simulink model "gm_uz_pmsm_model_6LUT_pd"  (R2023a)
settings: Solver=FixedStepAuto  StartTime=0.0  StopTime=0.05  RelTol=1e-3
PreLoadFcn:
  | uz_pmsm_model_init_parameter
PostLoadFcn:
  | % Import the data from Excel for a lookup table
  | FluxMapData = readtable('C:\Users\Philipp\ultrazohm\ultrazohm_sw\ip_cores\uz_pmsm_model\FluxMapData_2023-05-26_13-07-57.csv');
  | % Row indices for lookup table
  | d_current_in_d_axis = FluxMapData(8:27,1:end);
  | % Column indices for lookup table
  | q_current_in_d_axis = FluxMapData(29:48,1:end);
  | % Output values for lookup table
  | d_Flux_d_axis = FluxMapData(50:69,1:end);
undefined symbols (not defined in the file or in its folder): d_current_d_Flux, d_current_q_Flux, entkopplung_dynamic, entkopplung_linear, entkopplung_static, Flux_d, Flux_q, friction_coefficient, inertia, k_i_d, k_p_d, k_p_q, Ki_Bo_d, Ki_Bo_q, Kp_Bo_d, Kp_Bo_q, L_d, L_q, Ldd, Ldq, Lqd, Lqq, parameter_nachfuerung, polepair, praediktion_entkopplung_nonlinear, psi_pm, q_current_d_Flux, q_current_q_Flux, R_1, simulate_mechanical, simulate_nonlinear_modell, simulate_open_loop, static_friction_torque, tau_sum, ts, ts_regler
libraries: hdlmdlgenlib x5, slpidlib x4
(part 1 of 2)
settings Model: Creator=ts  LastModifiedBy=Philipp
settings SolverCC: AlgebraicLoopSolver=TrustRegion  AutoInsertRateTranBlk=on
settings DataIOCC: LimitDataPoints=on  SaveOutput=off  SaveTime=off
settings OptimizationCC: BlockReduction=off  ConditionallyExecuteInputs=off  DefaultParameterBehavior=Inlined  LifeSpan=inf
settings DebuggingCC: AlgebraicLoopMsg=error  InheritedTsInSrcMsg=none  SingleTaskRateTransMsg=error  UnconnectedInputMsg=warning  UnconnectedOutputMsg=warning  UnconnectedLineMsg=warning  AllowSymbolicDim=off  StrictBusMsg=ErrorOnBusTreatedAsVector  SFUnexpectedBacktrackingDiag=warning  SFNoUnconditionalDefaultTransitionDiag=warning  SFExecutionAtInitializationDiag=none  ArithmeticOperatorsInVariantConditions=warning
settings HardwareCC: ProdBitPerPointer=32  ProdBitPerSizeT=32  ProdBitPerPtrDiffT=32  ProdLargestAtomicFloat=None  ProdIntDivRoundTo=Undefined  ProdEndianess=Unspecified  ProdWordSize=32  ProdHWDeviceType=ASIC/FPGA->ASIC/FPGA  ProdEqTarget=off
settings ModelReferenceCC: EnableRefExpFcnMdlSchedulingChecks=on
settings SFSimCC: SimUseLocalCustomCode=off  CustomCodeUndefinedFunction=UseInterfaceOnly
settings RTWCC: RTWUseLocalCustomCode=off  DLArmComputeVersion=19.05
settings CodeAppCC: StateflowObjectComments=on
settings GRTTargetCC: TargetLangStandard=C89/C90 (ANSI)
settings ConfigComp: CovScope=ReferencedModels  CovMetricSettings=dw  CovSaveCumulativeToWorkspaceVar=on  CovSaveSingleToWorkspaceVar=on  CovExternalEMLEnable=off  CovSFcnEnable=off

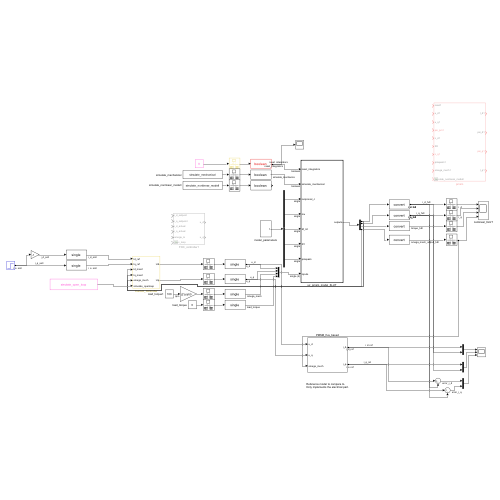
[thumbnail: Simulink's stored preview of the top-level diagram]
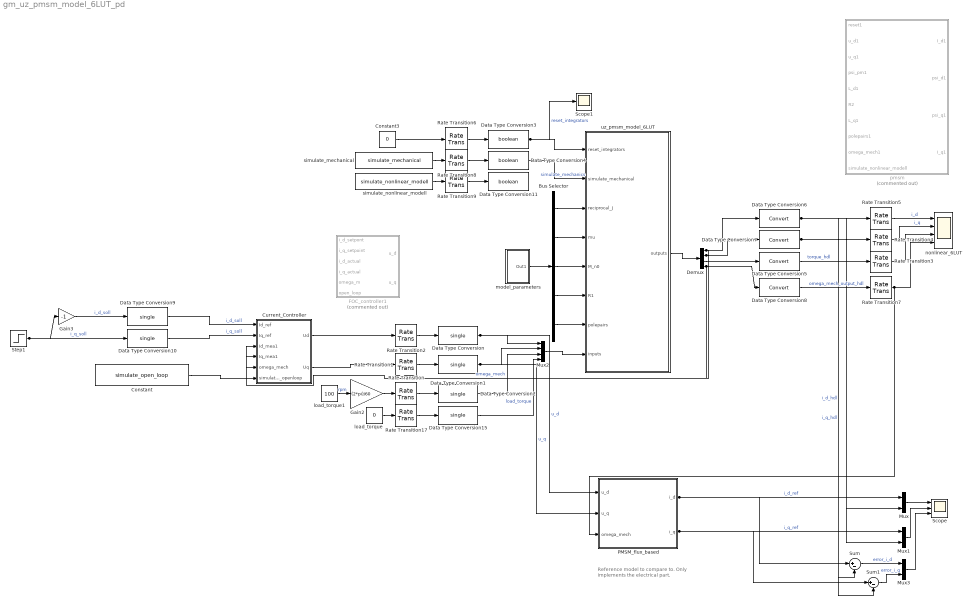
== system gm_uz_pmsm_model_6LUT_pd ==
  note: Reference model to compare to.
      | Only implements the electrical part.
  Bus Selector : BusSelector  OutputSignals=1_J,mu,M_R0,R_1,polepair
  Constant : Constant  Value=simulate_open_loop
  Constant3 : Constant  Value=0
  Current_Controller : Subsystem
  Data Type Conversion{,1..2,9..10,15} (6 alike) : DataTypeConversion  OutDataTypeStr=single  SaturateOnIntegerOverflow=off  RndMeth=Floor
  Data Type Conversion11 : DataTypeConversion  OutDataTypeStr=boolean  SaturateOnIntegerOverflow=off  RndMeth=Floor
  Data Type Conversion3 : DataTypeConversion  OutDataTypeStr=boolean  SaturateOnIntegerOverflow=off  RndMeth=Floor
  Data Type Conversion4 : DataTypeConversion  OutDataTypeStr=boolean  SaturateOnIntegerOverflow=off  RndMeth=Floor
  Data Type Conversion{5..8} (4 alike) : DataTypeConversion  SaturateOnIntegerOverflow=off  RndMeth=Floor
  Demux : Demux
  FOC_controller1 : Subsystem  Commented=on
  Gain2 : Gain  Gain=(2*pi)/60
  Gain3 : Gain  Gain=-1
  Mux : Mux  Inputs=2
  Mux1 : Mux  Inputs=2
  Mux2 : Mux
  Mux3 : Mux  Inputs=2
  PMSM_flux_based : Subsystem
  Rate Transition{,1..2,6,8..9,17} (7 alike) : RateTransition  OutPortSampleTime=ts
  Rate Transition{3..5,7} (4 alike) : RateTransition
  Scope : Scope  NumInputPorts=3
  Scope1 : Scope
  Step1 : Step  Time=0.025
  Sum : Sum  Inputs=|+-
  Sum1 : Sum  Inputs=|+-
  load_torque : Constant  Value=0
  load_torque1 : Constant  Value=100
  model_parameters : Subsystem
  nonlinear_6LUT : Scope  NumInputPorts=4
  pmsm : Subsystem  Commented=on
  simulate_mechanical : Constant  Value=simulate_mechanical
  simulate_nonlinear_modell : Constant  Value=simulate_nonlinear_modell
  uz_pmsm_model_6LUT : Subsystem  TreatAsAtomicUnit=on
  wires:
  Rate Transition9/1 -> Data Type Conversion11/1
  simulate_nonlinear_modell/1 -> Rate Transition9/1
  load_torque1/1 -> Gain2/1  "rpm"
  Constant/1 -> Current_Controller/6(simulate_openloop)
  Gain2/1 -> Rate Transition/1
  Current_Controller/2(Uq) -> Rate Transition1/1
  Current_Controller/1(Ud) -> Rate Transition2/1
  Data Type Conversion10/1 -> Current_Controller/2(Iq_ref)  "i_q_soll"
  Data Type Conversion9/1 -> Current_Controller/1(Id_ref)  "i_d_soll"
  uz_pmsm_model_6LUT/1(outputs) -> Demux/1
  Mux2/1 -> uz_pmsm_model_6LUT/8(inputs)
  Data Type Conversion2/1 -> Mux2/3  "omega_mech"
  Data Type Conversion15/1 -> Mux2/4  "load_torque"
  Data Type Conversion1/1 -> Mux2/2, PMSM_flux_based/2(u_q)  "u_q"
  Data Type Conversion/1 -> Mux2/1, PMSM_flux_based/1(u_d)  "u_d"
  Demux/2 -> Data Type Conversion7/1, Current_Controller/4(Iq_mea1)
  Demux/4 -> Data Type Conversion8/1, Current_Controller/5(omega_mech)
  Demux/1 -> Data Type Conversion6/1, Current_Controller/3(Id_mea1)
  Gain3/1 -> Data Type Conversion9/1  "i_d_soll"
  Demux/3 -> Data Type Conversion5/1
  Step1/1 -> Data Type Conversion10/1, Gain3/1  "i_q_soll"
  Mux3/1 -> Scope/3
  Sum1/1 -> Mux3/2  "error_i_q"
  Sum/1 -> Mux3/1  "error_i_d"
  model_parameters/1(Out1) -> Bus Selector/1
  Bus Selector/5 -> uz_pmsm_model_6LUT/7(polepairs)
  Bus Selector/4 -> uz_pmsm_model_6LUT/6(R1)
  Bus Selector/3 -> uz_pmsm_model_6LUT/5(M_n0)
  Bus Selector/2 -> uz_pmsm_model_6LUT/4(mu)
  Bus Selector/1 -> uz_pmsm_model_6LUT/3(reciprocal_J)
  Rate Transition7/1 -> nonlinear_6LUT/4, PMSM_flux_based/3(omega_mech)
  Data Type Conversion8/1 -> Rate Transition7/1  "omega_mech_output_hdl"
  PMSM_flux_based/1(i_d) -> Sum/1, Mux/1  "i_d_ref"
  PMSM_flux_based/2(i_q) -> Sum1/1, Mux1/1  "i_q_ref"
  Mux1/1 -> Scope/2
  Mux/1 -> Scope/1
  Rate Transition17/1 -> Data Type Conversion15/1
  load_torque/1 -> Rate Transition17/1
  Data Type Conversion4/1 -> uz_pmsm_model_6LUT/2(simulate_mechanical)  "simulate_mechanics"
  Data Type Conversion3/1 -> uz_pmsm_model_6LUT/1(reset_integrators), Scope1/1  "reset_integrators"
  simulate_mechanical/1 -> Rate Transition8/1
  Rate Transition8/1 -> Data Type Conversion4/1
  Constant3/1 -> Rate Transition6/1
  Rate Transition6/1 -> Data Type Conversion3/1
  Rate Transition3/1 -> nonlinear_6LUT/3
  Rate Transition5/1 -> nonlinear_6LUT/1  "i_d"
  Rate Transition4/1 -> nonlinear_6LUT/2  "i_q"
  Data Type Conversion5/1 -> Rate Transition3/1  "torque_hdl"
  Data Type Conversion7/1 -> Sum1/2, Mux1/2, Rate Transition4/1  "i_q_hdl"
  Data Type Conversion6/1 -> Rate Transition5/1, Sum/2, Mux/2  "i_d_hdl"
  Rate Transition2/1 -> Data Type Conversion/1
  Rate Transition1/1 -> Data Type Conversion1/1
  Rate Transition/1 -> Data Type Conversion2/1

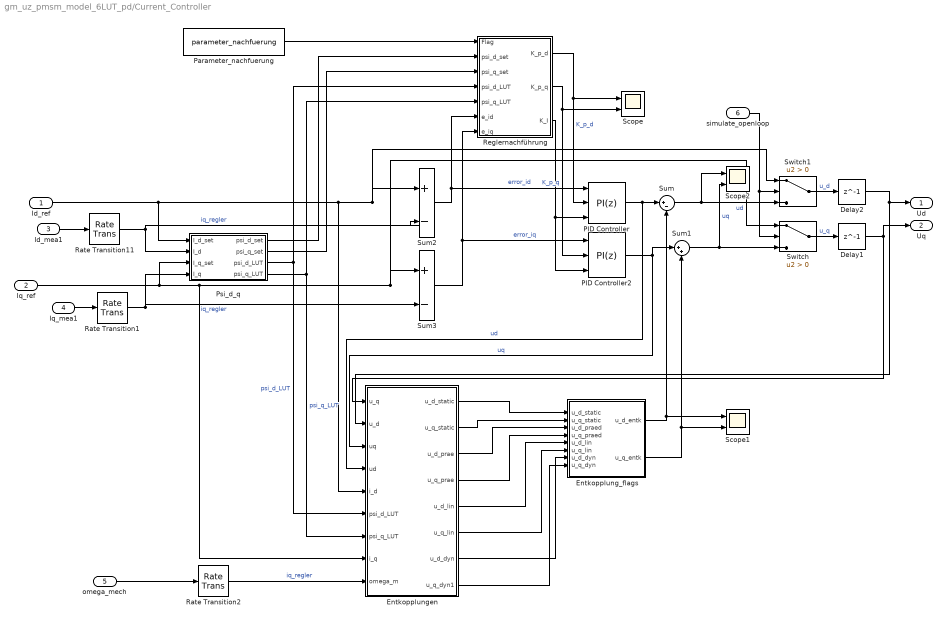
== system gm_uz_pmsm_model_6LUT_pd/Current_Controller ==
  Id_ref : Inport
  Iq_ref : Inport  Port=2
  Id_mea1 : Inport  Port=3
  Iq_mea1 : Inport  Port=4
  omega_mech : Inport  Port=5
  simulate_openloop : Inport  Port=6
  Delay1 : Delay  DelayLength=1
  Delay2 : Delay  DelayLength=1
  Entkopplung_flags : Subsystem
  Entkopplungen : Subsystem
  PID Controller : slpidlib/PID Controller  Controller=PI  Form=Parallel  TimeDomain=Discrete-time  UseExternalTs=off  SampleTime=-1  IntegratorMethod=Forward Euler  FilterMethod=Forward Euler  ControllerParametersSource=external  P=Kp_Bo_d  I=Ki_Bo_d  UseKiTs=off  D=0  N=100  UseFilter=on  TunerSelectOption=Transfer Function Based (PID Tuner App)  InitialConditionSource=internal  InitialConditionForIntegrator=0  InitialConditionForFilter=0  DifferentiatorICPrevScaledInput=0  ExternalReset=none  TrackingMode=off  Kt=1  LimitOutput=off  SatLimitsSource=internal  UpperSaturationLimit=48  LowerSaturationLimit=-48  LinearizeAsGain=off  AntiWindupMode=clamping  Kb=1  LimitIntegrator=off  UpperIntegratorSaturationLimit=48  LowerIntegratorSaturationLimit=-48  POutMin=[]  POutMax=[]  IOutMin=[]  IOutMax=[]  DOutMin=[]  DOutMax=[]  NOutMin=[]  NOutMax=[]  SumOutMin=[]  SumOutMax=[]  SaturationOutMin=[]  SaturationOutMax=[]  PParamMin=[]  PParamMax=[]  IParamMin=[]  IParamMax=[]  DParamMin=[]  DParamMax=[]  NParamMin=[]  NParamMax=[]  KbParamMin=[]  KbParamMax=[]  KtParamMin=[]  KtParamMax=[]  KbOutMin=[]  KbOutMax=[]  KtOutMin=[]  KtOutMax=[]  IntegratorOutMin=[]  IntegratorOutMax=[]  FilterOutMin=[]  FilterOutMax=[]  SumI1OutMin=[]  SumI1OutMax=[]  SumI2OutMin=[]  SumI2OutMax=[]  SumI3OutMin=[]  SumI3OutMax=[]  SumI4OutMin=[]  SumI4OutMax=[]  SumDOutMin=[]  SumDOutMax=[]  DifferentiatorOutMin=[]  DifferentiatorOutMax=[]  FilterDiffOutCoefMin=[]  FilterDiffOutCoefMax=[]  ReciprocalOutMin=[]  ReciprocalOutMax=[]  SumDenOutMin=[]  SumDenOutMax=[]  SumNumOutMin=[]  SumNumOutMax=[]  DivideOutMin=[]  DivideOutMax=[]  UdiffTsProdOutMin=[]  UdiffTsProdOutMax=[]  NTsProdOutMin=[]  NTsProdOutMax=[]  UintegralTsProdOutMin=[]  UintegralTsProdOutMax=[]  UngainTsProdOutMin=[]  UngainTsProdOutMax=[]  ClampingZeroOutDataTypeStr=Inherit: Inherit via back propagation  ClampingZeroOutMin=[]  ClampingZeroOutMax=[]  FilterDenConstantOutDataTypeStr=Inherit: Inherit via back propagation  FilterDenConstantOutMin=[]  FilterDenConstantOutMax=[]  PCopyOutDataTypeStr=Inherit: Inherit via back propagation  PCopyOutMin=[]  PCopyOutMax=[]  NCopyOutDataTypeStr=Inherit: Inherit via back propagation  NCopyOutMin=[]  NCopyOutMax=[]  IntegratorContinuousStateAttributes=''  IntegratorStateMustResolveToSignalObject=off  IntegratorRTWStateStorageClass=Auto  FilterContinuousStateAttributes=''  FilterStateMustResolveToSignalObject=off  FilterRTWStateStorageClass=Auto  ParallelPVariant=ExternalParameters  IdealPVariant=Disabled  IVariant=ExternalParameters  DVariant=Disabled  IntegratorVariant=Discrete  SatVariant=Disabled  AWVariant=Passthrough  PCopyVariant=Disabled  TRVariant=Disabled  FdbkBlocksVariant=Forward  IdealPFdbkVariant=Disabled  SatFdbkVariant=Disabled  DerivativeFilterVariant=Disabled  NVariant=Disabled  NCopyVariant=Disabled_SignalSpec  FilterICVariant=Disabled  IntegratorICVariant=InternalICs  ExternalResetVariant=Disabled  TRSumVariant=Passthrough  SumFdbkVariant=Disabled  SumVariant=Sum_PI  TsampFilterVariant=InternalTs  TsampNgainVariant=Passthrough  TsampIntegralVariant=Disabled_SignalSpec  ExternalSaturationOutDataTypeStr=Inherit: Same as second input
  PID Controller2 : slpidlib/PID Controller  Controller=PI  Form=Parallel  TimeDomain=Discrete-time  UseExternalTs=off  SampleTime=-1  IntegratorMethod=Forward Euler  FilterMethod=Forward Euler  ControllerParametersSource=external  P=Kp_Bo_q  I=Ki_Bo_q  UseKiTs=off  D=0  N=100  UseFilter=on  TunerSelectOption=Transfer Function Based (PID Tuner App)  InitialConditionSource=internal  InitialConditionForIntegrator=0  InitialConditionForFilter=0  DifferentiatorICPrevScaledInput=0  ExternalReset=none  TrackingMode=off  Kt=1  LimitOutput=off  SatLimitsSource=internal  UpperSaturationLimit=48  LowerSaturationLimit=-48  LinearizeAsGain=off  AntiWindupMode=clamping  Kb=1  LimitIntegrator=off  UpperIntegratorSaturationLimit=48  LowerIntegratorSaturationLimit=-48  POutMin=[]  POutMax=[]  IOutMin=[]  IOutMax=[]  DOutMin=[]  DOutMax=[]  NOutMin=[]  NOutMax=[]  SumOutMin=[]  SumOutMax=[]  SaturationOutMin=[]  SaturationOutMax=[]  PParamMin=[]  PParamMax=[]  IParamMin=[]  IParamMax=[]  DParamMin=[]  DParamMax=[]  NParamMin=[]  NParamMax=[]  KbParamMin=[]  KbParamMax=[]  KtParamMin=[]  KtParamMax=[]  KbOutMin=[]  KbOutMax=[]  KtOutMin=[]  KtOutMax=[]  IntegratorOutMin=[]  IntegratorOutMax=[]  FilterOutMin=[]  FilterOutMax=[]  SumI1OutMin=[]  SumI1OutMax=[]  SumI2OutMin=[]  SumI2OutMax=[]  SumI3OutMin=[]  SumI3OutMax=[]  SumI4OutMin=[]  SumI4OutMax=[]  SumDOutMin=[]  SumDOutMax=[]  DifferentiatorOutMin=[]  DifferentiatorOutMax=[]  FilterDiffOutCoefMin=[]  FilterDiffOutCoefMax=[]  ReciprocalOutMin=[]  ReciprocalOutMax=[]  SumDenOutMin=[]  SumDenOutMax=[]  SumNumOutMin=[]  SumNumOutMax=[]  DivideOutMin=[]  DivideOutMax=[]  UdiffTsProdOutMin=[]  UdiffTsProdOutMax=[]  NTsProdOutMin=[]  NTsProdOutMax=[]  UintegralTsProdOutMin=[]  UintegralTsProdOutMax=[]  UngainTsProdOutMin=[]  UngainTsProdOutMax=[]  ClampingZeroOutDataTypeStr=Inherit: Inherit via back propagation  ClampingZeroOutMin=[]  ClampingZeroOutMax=[]  FilterDenConstantOutDataTypeStr=Inherit: Inherit via back propagation  FilterDenConstantOutMin=[]  FilterDenConstantOutMax=[]  PCopyOutDataTypeStr=Inherit: Inherit via back propagation  PCopyOutMin=[]  PCopyOutMax=[]  NCopyOutDataTypeStr=Inherit: Inherit via back propagation  NCopyOutMin=[]  NCopyOutMax=[]  IntegratorContinuousStateAttributes=''  IntegratorStateMustResolveToSignalObject=off  IntegratorRTWStateStorageClass=Auto  FilterContinuousStateAttributes=''  FilterStateMustResolveToSignalObject=off  FilterRTWStateStorageClass=Auto  ParallelPVariant=ExternalParameters  IdealPVariant=Disabled  IVariant=ExternalParameters  DVariant=Disabled  IntegratorVariant=Discrete  SatVariant=Disabled  AWVariant=Passthrough  PCopyVariant=Disabled  TRVariant=Disabled  FdbkBlocksVariant=Forward  IdealPFdbkVariant=Disabled  SatFdbkVariant=Disabled  DerivativeFilterVariant=Disabled  NVariant=Disabled  NCopyVariant=Disabled_SignalSpec  FilterICVariant=Disabled  IntegratorICVariant=InternalICs  ExternalResetVariant=Disabled  TRSumVariant=Passthrough  SumFdbkVariant=Disabled  SumVariant=Sum_PI  TsampFilterVariant=InternalTs  TsampNgainVariant=Passthrough  TsampIntegralVariant=Disabled_SignalSpec  ExternalSaturationOutDataTypeStr=Inherit: Same as second input
  Parameter_nachfuerung : Constant  Value=parameter_nachfuerung
  Psi_d_q : Subsystem
  Rate Transition1 : RateTransition  OutPortSampleTime=ts_regler
  Rate Transition11 : RateTransition  OutPortSampleTime=ts_regler
  Rate Transition2 : RateTransition  OutPortSampleTime=ts_regler
  Reglernachführung : Subsystem
  Scope : Scope  NumInputPorts=2
  Scope1 : Scope  NumInputPorts=2
  Scope2 : Scope  NumInputPorts=2
  Sum : Sum  Inputs=|+-
  Sum1 : Sum  Inputs=|++
  Sum2 : Sum  Inputs=|+-
  Sum3 : Sum  Inputs=|+-
  Switch : Switch  Criteria=u2 > Threshold  SaturateOnIntegerOverflow=off  InputSameDT=off
  Switch1 : Switch  Criteria=u2 > Threshold  SaturateOnIntegerOverflow=off  InputSameDT=off
  Ud : Outport
  Uq : Outport  Port=2
  wires:
  Entkopplungen/8(u_q_dyn1) -> Entkopplung_flags/8(u_q_dyn)
  Entkopplungen/7(u_d_dyn) -> Entkopplung_flags/7(u_d_dyn)
  Delay1/1 -> Entkopplungen/1(u_q), Uq/1
  Delay2/1 -> Entkopplungen/2(u_d), Ud/1
  Rate Transition2/1 -> Entkopplungen/9(omega_m)  "iq_regler"
  Rate Transition1/1 -> Psi_d_q/4(I_q), Sum3/2  "iq_regler"
  Rate Transition11/1 -> Psi_d_q/2(I_d), Sum2/2  "iq_regler"
  Entkopplung_flags/2(u_q_entk) -> Sum1/2, Scope1/2
  Entkopplung_flags/1(u_d_entk) -> Sum/2, Scope1/1
  Entkopplungen/6(u_q_lin) -> Entkopplung_flags/6(u_q_lin)
  Entkopplungen/5(u_d_lin) -> Entkopplung_flags/5(u_d_lin)
  Entkopplungen/4(u_q_prae) -> Entkopplung_flags/4(u_q_praed)
  Entkopplungen/3(u_d_prae) -> Entkopplung_flags/3(u_d_praed)
  Entkopplungen/2(u_q_static) -> Entkopplung_flags/2(u_q_static)
  Entkopplungen/1(u_d_static) -> Entkopplung_flags/1(u_d_static)
  omega_mech/1 -> Rate Transition2/1
  Psi_d_q/2(psi_q_set) -> Reglernachführung/3(psi_q_set)
  Psi_d_q/1(psi_d_set) -> Reglernachführung/2(psi_d_set)
  Parameter_nachfuerung/1 -> Reglernachführung/1(Flag)
  Psi_d_q/4(psi_q_LUT) -> Entkopplungen/7(psi_q_LUT), Reglernachführung/5(psi_q_LUT)  "psi_q_LUT"
  Psi_d_q/3(psi_d_LUT) -> Entkopplungen/6(psi_d_LUT), Reglernachführung/4(psi_d_LUT)  "psi_d_LUT"
  Iq_mea1/1 -> Rate Transition1/1
  Id_mea1/1 -> Rate Transition11/1
  Reglernachführung/3(K_I) -> PID Controller/3, PID Controller2/3
  Reglernachführung/2(K_p_q) -> Scope/2, PID Controller2/2  "K_p_q"
  Reglernachführung/1(K_p_d) -> Scope/1, PID Controller/2  "K_p_d"
  simulate_openloop/1 -> Switch1/2, Switch/2
  Switch1/1 -> Delay2/1  "u_d"
  Switch/1 -> Delay1/1  "u_q"
  Id_ref/1 -> Switch1/1, Sum2/1, Entkopplungen/5(i_d), Psi_d_q/1(I_d_set)
  Iq_ref/1 -> Psi_d_q/3(I_q_set), Switch/1, Sum3/1, Entkopplungen/8(i_q)
  Sum1/1 -> Switch/3, Scope2/2  "uq"
  PID Controller2/1 -> Entkopplungen/3(uq), Sum1/1  "uq"
  PID Controller/1 -> Sum/1, Entkopplungen/4(ud)  "ud"
  Sum/1 -> Switch1/3, Scope2/1  "ud"
  Sum2/1 -> Reglernachführung/6(e_id), PID Controller/1  "error_id"
  Sum3/1 -> PID Controller2/1, Reglernachführung/7(e_iq)  "error_iq"

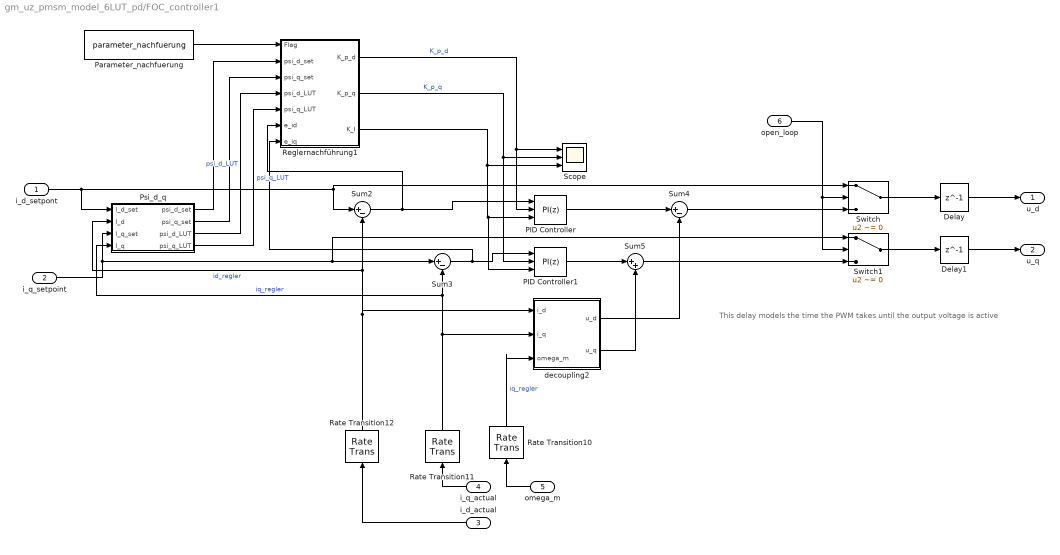
== system gm_uz_pmsm_model_6LUT_pd/FOC_controller1 ==
  note: This delay models the time the PWM takes until the output voltage is active
  i_d_setpont : Inport
  i_q_setpoint : Inport  Port=2
  i_d_actual : Inport  Port=3
  i_q_actual : Inport  Port=4
  omega_m : Inport  Port=5
  open_loop : Inport  Port=6
  Delay : Delay  DelayLength=1
  Delay1 : Delay  DelayLength=1
  PID Controller : slpidlib/PID Controller  Controller=PI  Form=Parallel  TimeDomain=Discrete-time  UseExternalTs=off  SampleTime=-1  IntegratorMethod=Forward Euler  FilterMethod=Forward Euler  ControllerParametersSource=external  P=k_p_d  I=k_i_d  UseKiTs=off  D=0  N=100  UseFilter=on  TunerSelectOption=Transfer Function Based (PID Tuner App)  InitialConditionSource=internal  InitialConditionForIntegrator=0  InitialConditionForFilter=0  DifferentiatorICPrevScaledInput=0  ExternalReset=none  TrackingMode=off  Kt=1  LimitOutput=off  SatLimitsSource=internal  UpperSaturationLimit=48  LowerSaturationLimit=-48  LinearizeAsGain=on  AntiWindupMode=clamping  Kb=1  LimitIntegrator=off  UpperIntegratorSaturationLimit=inf  LowerIntegratorSaturationLimit=-inf  POutMin=[]  POutMax=[]  IOutMin=[]  IOutMax=[]  DOutMin=[]  DOutMax=[]  NOutMin=[]  NOutMax=[]  SumOutMin=[]  SumOutMax=[]  SaturationOutMin=[]  SaturationOutMax=[]  PParamMin=[]  PParamMax=[]  IParamMin=[]  IParamMax=[]  DParamMin=[]  DParamMax=[]  NParamMin=[]  NParamMax=[]  KbParamMin=[]  KbParamMax=[]  KtParamMin=[]  KtParamMax=[]  KbOutMin=[]  KbOutMax=[]  KtOutMin=[]  KtOutMax=[]  IntegratorOutMin=[]  IntegratorOutMax=[]  FilterOutMin=[]  FilterOutMax=[]  SumI1OutMin=[]  SumI1OutMax=[]  SumI2OutMin=[]  SumI2OutMax=[]  SumI3OutMin=[]  SumI3OutMax=[]  SumI4OutMin=[]  SumI4OutMax=[]  SumDOutMin=[]  SumDOutMax=[]  DifferentiatorOutMin=[]  DifferentiatorOutMax=[]  FilterDiffOutCoefMin=[]  FilterDiffOutCoefMax=[]  ReciprocalOutMin=[]  ReciprocalOutMax=[]  SumDenOutMin=[]  SumDenOutMax=[]  SumNumOutMin=[]  SumNumOutMax=[]  DivideOutMin=[]  DivideOutMax=[]  UdiffTsProdOutMin=[]  UdiffTsProdOutMax=[]  NTsProdOutMin=[]  NTsProdOutMax=[]  UintegralTsProdOutMin=[]  UintegralTsProdOutMax=[]  UngainTsProdOutMin=[]  UngainTsProdOutMax=[]  ClampingZeroOutDataTypeStr=Inherit: Inherit via back propagation  ClampingZeroOutMin=[]  ClampingZeroOutMax=[]  FilterDenConstantOutDataTypeStr=Inherit: Inherit via back propagation  FilterDenConstantOutMin=[]  FilterDenConstantOutMax=[]  PCopyOutDataTypeStr=Inherit: Inherit via back propagation  PCopyOutMin=[]  PCopyOutMax=[]  NCopyOutDataTypeStr=Inherit: Inherit via back propagation  NCopyOutMin=[]  NCopyOutMax=[]  IntegratorContinuousStateAttributes=''  IntegratorStateMustResolveToSignalObject=off  IntegratorRTWStateStorageClass=Auto  FilterContinuousStateAttributes=''  FilterStateMustResolveToSignalObject=off  FilterRTWStateStorageClass=Auto  ParallelPVariant=ExternalParameters  IdealPVariant=Disabled  IVariant=ExternalParameters  DVariant=Disabled  IntegratorVariant=Discrete  SatVariant=Disabled  AWVariant=Passthrough  PCopyVariant=Disabled  TRVariant=Disabled  FdbkBlocksVariant=Forward  IdealPFdbkVariant=Disabled  SatFdbkVariant=Disabled  DerivativeFilterVariant=Disabled  NVariant=Disabled  NCopyVariant=Disabled_SignalSpec  FilterICVariant=Disabled  IntegratorICVariant=InternalICs  ExternalResetVariant=Disabled  TRSumVariant=Passthrough  SumFdbkVariant=Disabled  SumVariant=Sum_PI  TsampFilterVariant=InternalTs  TsampNgainVariant=Passthrough  TsampIntegralVariant=Disabled_SignalSpec  ExternalSaturationOutDataTypeStr=Inherit: Same as second input
  PID Controller1 : slpidlib/PID Controller  Controller=PI  Form=Parallel  TimeDomain=Discrete-time  UseExternalTs=off  SampleTime=-1  IntegratorMethod=Forward Euler  FilterMethod=Forward Euler  ControllerParametersSource=external  P=k_p_q  I=k_i_d  UseKiTs=off  D=0  N=100  UseFilter=on  TunerSelectOption=Transfer Function Based (PID Tuner App)  InitialConditionSource=internal  InitialConditionForIntegrator=0  InitialConditionForFilter=0  DifferentiatorICPrevScaledInput=0  ExternalReset=none  TrackingMode=off  Kt=1  LimitOutput=off  SatLimitsSource=internal  UpperSaturationLimit=48  LowerSaturationLimit=-48  LinearizeAsGain=on  AntiWindupMode=clamping  Kb=1  LimitIntegrator=off  UpperIntegratorSaturationLimit=inf  LowerIntegratorSaturationLimit=-inf  POutMin=[]  POutMax=[]  IOutMin=[]  IOutMax=[]  DOutMin=[]  DOutMax=[]  NOutMin=[]  NOutMax=[]  SumOutMin=[]  SumOutMax=[]  SaturationOutMin=[]  SaturationOutMax=[]  PParamMin=[]  PParamMax=[]  IParamMin=[]  IParamMax=[]  DParamMin=[]  DParamMax=[]  NParamMin=[]  NParamMax=[]  KbParamMin=[]  KbParamMax=[]  KtParamMin=[]  KtParamMax=[]  KbOutMin=[]  KbOutMax=[]  KtOutMin=[]  KtOutMax=[]  IntegratorOutMin=[]  IntegratorOutMax=[]  FilterOutMin=[]  FilterOutMax=[]  SumI1OutMin=[]  SumI1OutMax=[]  SumI2OutMin=[]  SumI2OutMax=[]  SumI3OutMin=[]  SumI3OutMax=[]  SumI4OutMin=[]  SumI4OutMax=[]  SumDOutMin=[]  SumDOutMax=[]  DifferentiatorOutMin=[]  DifferentiatorOutMax=[]  FilterDiffOutCoefMin=[]  FilterDiffOutCoefMax=[]  ReciprocalOutMin=[]  ReciprocalOutMax=[]  SumDenOutMin=[]  SumDenOutMax=[]  SumNumOutMin=[]  SumNumOutMax=[]  DivideOutMin=[]  DivideOutMax=[]  UdiffTsProdOutMin=[]  UdiffTsProdOutMax=[]  NTsProdOutMin=[]  NTsProdOutMax=[]  UintegralTsProdOutMin=[]  UintegralTsProdOutMax=[]  UngainTsProdOutMin=[]  UngainTsProdOutMax=[]  ClampingZeroOutDataTypeStr=Inherit: Inherit via back propagation  ClampingZeroOutMin=[]  ClampingZeroOutMax=[]  FilterDenConstantOutDataTypeStr=Inherit: Inherit via back propagation  FilterDenConstantOutMin=[]  FilterDenConstantOutMax=[]  PCopyOutDataTypeStr=Inherit: Inherit via back propagation  PCopyOutMin=[]  PCopyOutMax=[]  NCopyOutDataTypeStr=Inherit: Inherit via back propagation  NCopyOutMin=[]  NCopyOutMax=[]  IntegratorContinuousStateAttributes=''  IntegratorStateMustResolveToSignalObject=off  IntegratorRTWStateStorageClass=Auto  FilterContinuousStateAttributes=''  FilterStateMustResolveToSignalObject=off  FilterRTWStateStorageClass=Auto  ParallelPVariant=ExternalParameters  IdealPVariant=Disabled  IVariant=ExternalParameters  DVariant=Disabled  IntegratorVariant=Discrete  SatVariant=Disabled  AWVariant=Passthrough  PCopyVariant=Disabled  TRVariant=Disabled  FdbkBlocksVariant=Forward  IdealPFdbkVariant=Disabled  SatFdbkVariant=Disabled  DerivativeFilterVariant=Disabled  NVariant=Disabled  NCopyVariant=Disabled_SignalSpec  FilterICVariant=Disabled  IntegratorICVariant=InternalICs  ExternalResetVariant=Disabled  TRSumVariant=Passthrough  SumFdbkVariant=Disabled  SumVariant=Sum_PI  TsampFilterVariant=InternalTs  TsampNgainVariant=Passthrough  TsampIntegralVariant=Disabled_SignalSpec  ExternalSaturationOutDataTypeStr=Inherit: Same as second input
  Parameter_nachfuerung : Constant  Value=parameter_nachfuerung
  Psi_d_q : Subsystem
  Rate Transition10 : RateTransition  OutPortSampleTime=ts_regler
  Rate Transition11 : RateTransition  OutPortSampleTime=ts_regler
  Rate Transition12 : RateTransition  OutPortSampleTime=ts_regler
  Reglernachführung1 : Subsystem
  Scope : Scope  NumInputPorts=3
  Sum2 : Sum  Inputs=|+-
  Sum3 : Sum  Inputs=|+-
  Sum4 : Sum  Inputs=|+-
  Sum5 : Sum  Inputs=|++
  Switch : Switch  Criteria=u2 ~= 0  SaturateOnIntegerOverflow=off  InputSameDT=off
  Switch1 : Switch  Criteria=u2 ~= 0  SaturateOnIntegerOverflow=off  InputSameDT=off
  decoupling2 : Subsystem
  u_d : Outport
  u_q : Outport  Port=2
  wires:
  Parameter_nachfuerung/1 -> Reglernachführung1/1(Flag)
  Psi_d_q/4(psi_q_LUT) -> Reglernachführung1/5(psi_q_LUT)  "psi_q_LUT"
  Psi_d_q/3(psi_d_LUT) -> Reglernachführung1/4(psi_d_LUT)  "psi_d_LUT"
  Psi_d_q/2(psi_q_set) -> Reglernachführung1/3(psi_q_set)
  Psi_d_q/1(psi_d_set) -> Reglernachführung1/2(psi_d_set)
  Reglernachführung1/3(K_I) -> Scope/3, PID Controller/3, PID Controller1/3
  Reglernachführung1/2(K_p_q) -> Scope/2, PID Controller1/2  "K_p_q"
  Reglernachführung1/1(K_p_d) -> Scope/1, PID Controller/2  "K_p_d"
  Delay1/1 -> u_q/1
  Delay/1 -> u_d/1
  Switch1/1 -> Delay1/1
  Switch/1 -> Delay/1
  decoupling2/2(u_q) -> Sum5/2
  decoupling2/1(u_d) -> Sum4/2
  Rate Transition10/1 -> decoupling2/3(omega_m)  "iq_regler"
  open_loop/1 -> Switch/2, Switch1/2
  i_q_setpoint/1 -> Psi_d_q/3(I_q_set), Sum3/1, Switch1/1
  Rate Transition11/1 -> decoupling2/2(i_q), Psi_d_q/4(I_q), Sum3/2  "iq_regler"
  Rate Transition12/1 -> decoupling2/1(i_d), Sum2/2, Psi_d_q/2(I_d)  "id_regler"
  i_q_actual/1 -> Rate Transition11/1
  Sum3/1 -> PID Controller1/1, Reglernachführung1/7(e_iq)
  omega_m/1 -> Rate Transition10/1
  Sum5/1 -> Switch1/3
  Sum2/1 -> PID Controller/1, Reglernachführung1/6(e_id)
  i_d_setpont/1 -> Psi_d_q/1(I_d_set), Switch/1, Sum2/1
  i_d_actual/1 -> Rate Transition12/1
  Sum4/1 -> Switch/3
  PID Controller1/1 -> Sum5/1
  PID Controller/1 -> Sum4/1

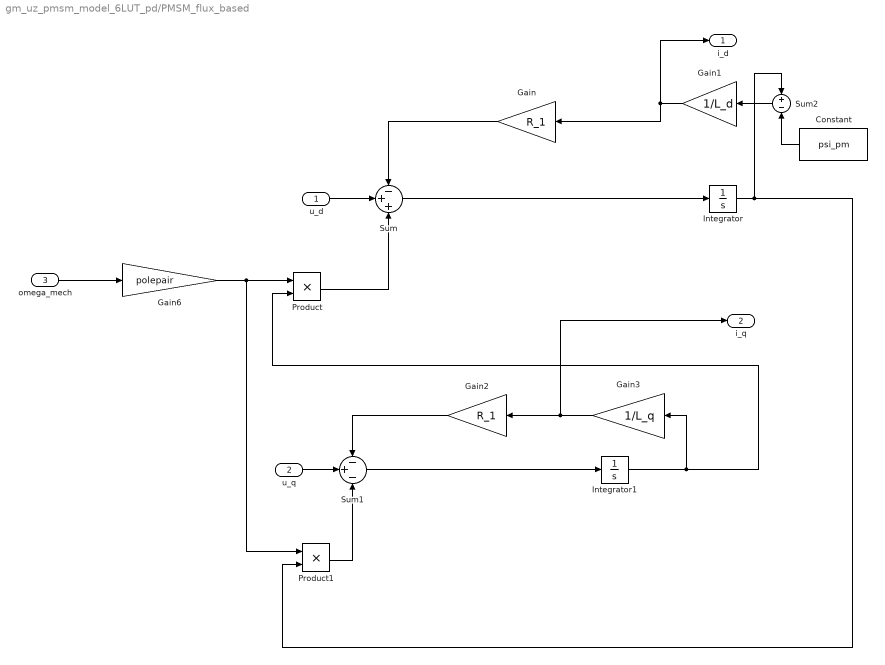
== system gm_uz_pmsm_model_6LUT_pd/PMSM_flux_based ==
  u_d : Inport
  u_q : Inport  Port=2
  omega_mech : Inport  Port=3
  Constant : Constant  Value=psi_pm
  Gain : Gain  Gain=R_1
  Gain1 : Gain  Gain=1/L_d
  Gain2 : Gain  Gain=R_1
  Gain3 : Gain  Gain=1/L_q
  Gain6 : Gain  Gain=polepair
  Integrator : Integrator
  Integrator1 : Integrator
  Product : Product
  Product1 : Product
  Sum : Sum  Inputs=-++
  Sum1 : Sum  Inputs=-+-
  Sum2 : Sum  Inputs=+-
  i_d : Outport
  i_q : Outport  Port=2
  wires:
  omega_mech/1 -> Gain6/1
  Gain3/1 -> Gain2/1, i_q/1
  Gain2/1 -> Sum1/1
  Sum1/1 -> Integrator1/1
  Product1/1 -> Sum1/3
  Integrator1/1 -> Product/2, Gain3/1
  Product/1 -> Sum/3
  Gain6/1 -> Product/1, Product1/1
  Gain1/1 -> i_d/1, Gain/1
  Sum2/1 -> Gain1/1
  Constant/1 -> Sum2/2
  Integrator/1 -> Sum2/1, Product1/2
  Gain/1 -> Sum/1
  Sum/1 -> Integrator/1
  u_q/1 -> Sum1/2
  u_d/1 -> Sum/2

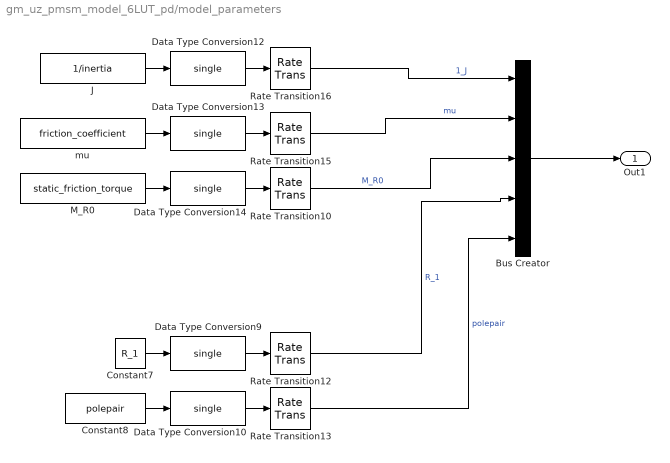
== system gm_uz_pmsm_model_6LUT_pd/model_parameters ==
  Bus Creator : BusCreator  Inputs=5
  Constant7 : Constant  Value=R_1
  Constant8 : Constant  Value=polepair
  Data Type Conversion{9..10,12..14} (5 alike) : DataTypeConversion  OutDataTypeStr=single  SaturateOnIntegerOverflow=off  RndMeth=Floor
  J : Constant  Value=1/inertia
  M_R0 : Constant  Value=static_friction_torque
  Rate Transition{10,12..13,15..16} (5 alike) : RateTransition  OutPortSampleTime=ts
  mu : Constant  Value=friction_coefficient
  Out1 : Outport
  wires:
  Constant7/1 -> Data Type Conversion9/1
  Data Type Conversion13/1 -> Rate Transition15/1
  M_R0/1 -> Data Type Conversion14/1
  mu/1 -> Data Type Conversion13/1
  Data Type Conversion10/1 -> Rate Transition13/1
  J/1 -> Data Type Conversion12/1
  Rate Transition15/1 -> Bus Creator/2  "mu"
  Data Type Conversion9/1 -> Rate Transition12/1
  Constant8/1 -> Data Type Conversion10/1
  Bus Creator/1 -> Out1/1
  Rate Transition13/1 -> Bus Creator/5  "polepair"
  Rate Transition16/1 -> Bus Creator/1  "1_J"
  Rate Transition12/1 -> Bus Creator/4  "R_1"
  Data Type Conversion14/1 -> Rate Transition10/1
  Rate Transition10/1 -> Bus Creator/3  "M_R0"
  Data Type Conversion12/1 -> Rate Transition16/1

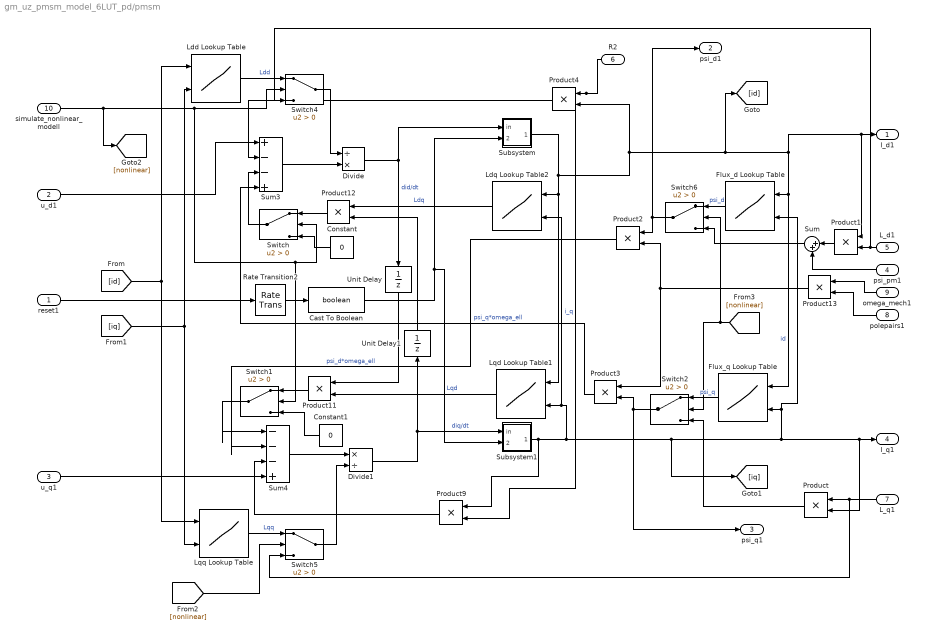
== system gm_uz_pmsm_model_6LUT_pd/pmsm ==
  reset1 : Inport
  u_d1 : Inport  Port=2
  u_q1 : Inport  Port=3
  psi_pm1 : Inport  Port=4
  L_d1 : Inport  Port=5
  R2 : Inport  Port=6
  L_q1 : Inport  Port=7
  polepairs1 : Inport  Port=8
  omega_mech1 : Inport  Port=9
  simulate_nonlinear_modell : Inport  Port=10
  Cast To Boolean : DataTypeConversion  OutDataTypeStr=boolean  SaturateOnIntegerOverflow=off  RndMeth=Floor
  Constant : Constant  Value=0  SampleTime=ts
  Constant1 : Constant  Value=0  SampleTime=ts
  Divide : Product  Inputs=/*
  Divide1 : Product  Inputs=*/
  Flux_d Lookup Table : Lookup_n-D  BreakpointsForDimension1=d_current_d_Flux  BreakpointsForDimension2=q_current_d_Flux  BreakpointsForDimension3=[5, 7]  Table=Flux_d  InternalRulePriority=Speed  RndMeth=Simplest
      settings: InputPortMap=u0,u1
  Flux_q Lookup Table : Lookup_n-D  BreakpointsForDimension1=d_current_q_Flux  BreakpointsForDimension2=q_current_q_Flux  BreakpointsForDimension3=[5, 7]  Table=Flux_q  InternalRulePriority=Speed  RndMeth=Simplest
      settings: InputPortMap=u0,u1
  Ldd Lookup Table : Lookup_n-D  BreakpointsForDimension1=d_current_q_Flux  BreakpointsForDimension2=q_current_q_Flux  BreakpointsForDimension3=[5, 7]  Table=Ldd  InternalRulePriority=Speed  RndMeth=Simplest
      settings: InputPortMap=u0,u1
  Ldq Lookup Table2 : Lookup_n-D  BreakpointsForDimension1=d_current_q_Flux  BreakpointsForDimension2=q_current_q_Flux  BreakpointsForDimension3=[5, 7]  Table=Ldq  InternalRulePriority=Speed  RndMeth=Simplest
      settings: InputPortMap=u0,u1
  Lqd Lookup Table1 : Lookup_n-D  BreakpointsForDimension1=d_current_q_Flux  BreakpointsForDimension2=q_current_q_Flux  BreakpointsForDimension3=[5, 7]  Table=Lqd  InternalRulePriority=Speed  RndMeth=Simplest
      settings: InputPortMap=u0,u1
  Lqq Lookup Table : Lookup_n-D  BreakpointsForDimension1=d_current_q_Flux  BreakpointsForDimension2=q_current_q_Flux  BreakpointsForDimension3=[5, 7]  Table=Lqq  InternalRulePriority=Speed  RndMeth=Simplest
      settings: InputPortMap=u0,u1
  Product{,1..4,9,11..13} (9 alike) : Product
  Rate Transition2 : RateTransition  OutPortSampleTime=ts
  Subsystem : Subsystem
  Subsystem1 : Subsystem
  Sum : Sum  Inputs=|++
  Sum3 : Sum  Inputs=|+--+
  Sum4 : Sum  Inputs=|---+
  Switch{,1..2,4..6} (6 alike) : Switch  Criteria=u2 > Threshold  SaturateOnIntegerOverflow=off  InputSameDT=off
  Unit Delay : UnitDelay  SampleTime=-1  HasFrameUpgradeWarning=on
  Unit Delay1 : UnitDelay  SampleTime=-1  HasFrameUpgradeWarning=on
  I_d1 : Outport
  psi_d1 : Outport  Port=2
  psi_q1 : Outport  Port=3
  I_q1 : Outport  Port=4
  wires:
  [nonlinear] -> Switch6/2, Switch2/2
  [nonlinear] -> Switch5/2
  simulate_nonlinear_modell/1 -> Switch4/2, Switch1/2, Switch/2, [nonlinear]
  Sum/1 -> Switch6/3
  Product1/1 -> Sum/1
  Switch6/1 -> Product2/1, psi_d1/1
  Flux_d Lookup Table/1 -> Switch6/1  "psi_d"
  Switch5/1 -> Divide1/2
  Lqq Lookup Table/1 -> Switch5/1  "Lqq"
  Switch4/1 -> Divide/1
  Ldd Lookup Table/1 -> Switch4/1  "Ldd"
  Product/1 -> Switch2/3
  Switch2/1 -> Product3/2, psi_q1/1
  Flux_q Lookup Table/1 -> Switch2/1  "psi_q"
  L_q1/1 -> Product/1, Switch5/3
  Constant1/1 -> Switch1/3
  Switch1/1 -> Sum4/1
  Product11/1 -> Switch1/1
  Constant/1 -> Switch/3
  Switch/1 -> Sum3/3
  Product12/1 -> Switch/1
  Ldq Lookup Table2/1 -> Product12/1  "Ldq"
  Lqd Lookup Table1/1 -> Product11/2  "Lqd"
  Unit Delay1/1 -> Product12/2
  Unit Delay/1 -> Product11/1
  Product2/1 -> Sum4/2  "psi_d*omega_ell"
  Product4/1 -> Sum3/2
  Product3/1 -> Sum3/4  "psi_q*omega_ell"
  [iq] -> Lqq Lookup Table/2, Ldd Lookup Table/2
  Subsystem1/1(outt) -> Product9/1, Lqd Lookup Table1/2, Ldq Lookup Table2/2, Flux_d Lookup Table/2, Flux_q Lookup Table/2, Product/2, I_q1/1, [iq]  "i_q"
  psi_pm1/1 -> Sum/2
  [id] -> Ldd Lookup Table/1, Lqq Lookup Table/1
  Subsystem/1(outt) -> [id], I_d1/1, Product1/1, Flux_q Lookup Table/1, Flux_d Lookup Table/1, Product4/2, Ldq Lookup Table2/1, Lqd Lookup Table1/1  "id"
  R2/1 -> Product4/1, Product9/2
  Rate Transition2/1 -> Cast To Boolean/1
  reset1/1 -> Rate Transition2/1
  u_d1/1 -> Sum3/1
  Cast To Boolean/1 -> Subsystem1/2(reset), Subsystem/2(reset)
  Product9/1 -> Sum4/3
  Sum3/1 -> Divide/2
  Divide/1 -> Subsystem/1(in), Unit Delay/1  "did/dt"
  Product13/1 -> Product2/2, Product3/1
  polepairs1/1 -> Product13/2
  Divide1/1 -> Subsystem1/1(in), Unit Delay1/1  "diq/dt"
  L_d1/1 -> Product1/2, Switch4/3
  omega_mech1/1 -> Product13/1
  u_q1/1 -> Sum4/4
  Sum4/1 -> Divide1/1

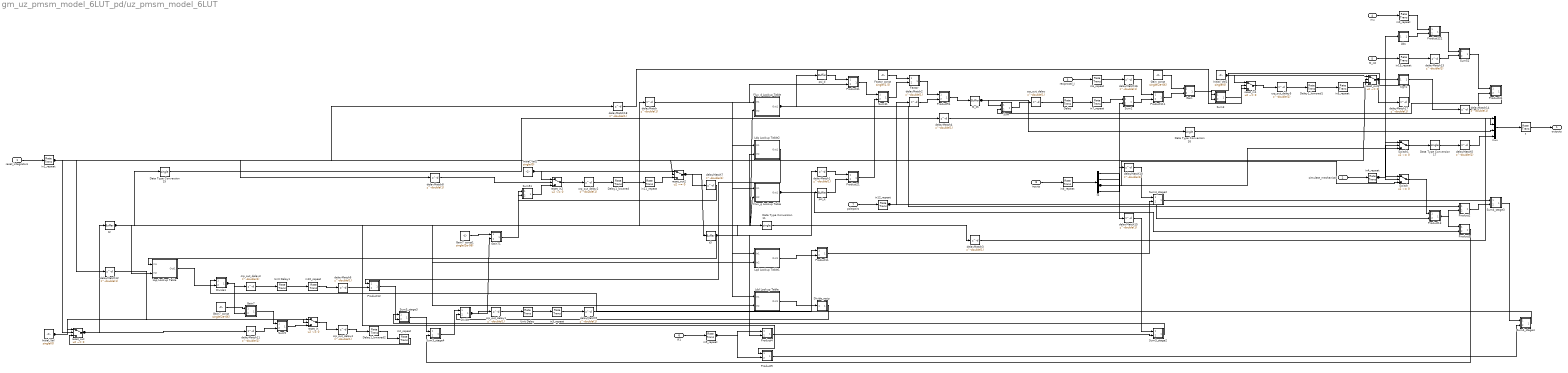
== system gm_uz_pmsm_model_6LUT_pd/uz_pmsm_model_6LUT ==
  reset_integrators : Inport  OutDataTypeStr=boolean  PortDimensions=1  SampleTime=2e-06
  simulate_mechanical : Inport  Port=2  OutDataTypeStr=boolean  PortDimensions=1  SampleTime=2e-06
  reciprocal_J : Inport  Port=3  OutDataTypeStr=single  PortDimensions=1  SampleTime=2e-06
  mu : Inport  Port=4  OutDataTypeStr=single  PortDimensions=1  SampleTime=2e-06
  M_n0 : Inport  Port=5  OutDataTypeStr=single  PortDimensions=1  SampleTime=2e-06
  R1 : Inport  Port=6  OutDataTypeStr=single  PortDimensions=1  SampleTime=2e-06
  polepairs : Inport  Port=7  OutDataTypeStr=single  PortDimensions=1  SampleTime=2e-06
  inputs : Inport  Port=8  OutDataTypeStr=single  PortDimensions=[4]  SampleTime=2e-06
  Abs : Subsystem
      mask Display: disp('NFP\nabs');
  Data Type Conversion{11,15..17} (4 alike) : DataTypeConversion  OutDataTypeStr=single
  Delay : RateTransition  OutPortSampleTimeOpt=Multiple of input port sample time  OutPortSampleTimeMultiple=200
  Delay1_lowered : RateTransition  OutPortSampleTimeOpt=Multiple of input port sample time  OutPortSampleTimeMultiple=200
  Delay1_lowered1 : RateTransition  OutPortSampleTimeOpt=Multiple of input port sample time  OutPortSampleTimeMultiple=200
  Delay1_lowered2 : RateTransition  OutPortSampleTimeOpt=Multiple of input port sample time  OutPortSampleTimeMultiple=200
  Divide : Subsystem
      mask Display: disp('NFP\nmul');
  Divide1 : Subsystem
      mask Display: disp('NFP\nmul');
  Divide_recip : Subsystem
      mask Display: disp('NFP\nmath');
  Factor : Subsystem
      mask Display: disp('NFP\nmul');
  Factor_const : Constant  Value=single(1.5)  OutDataTypeStr=single  SampleTime=1e-08
  Flux_d Lookup Table : Subsystem
  Flux_q Lookup Table : Subsystem
  Gain : Subsystem
      mask Display: disp('NFP\nmul');
  Gain7 : Subsystem
      mask Display: disp('NFP\nmul');
  Gain71 : Subsystem
      mask Display: disp('NFP\nmul');
  Gain7_const : Constant  Value=single(2e-06)  OutDataTypeStr=single  SampleTime=1e-08
  Gain7_const1 : Constant  Value=single(2e-06)  OutDataTypeStr=single  SampleTime=1e-08
  Gain_const : Constant  Value=single(2e-06)  OutDataTypeStr=single  SampleTime=1e-08
  Initial_Val : Constant  Value=single(0)  OutDataTypeStr=single  SampleTime=1e-08
  Initial_Val1 : Constant  Value=single(0)  OutDataTypeStr=single  SampleTime=1e-08
  Initial_Val2 : Constant  Value=single(0)  OutDataTypeStr=single  SampleTime=1e-08
  Ldd Lookup Table : Subsystem
  Ldq Lookup Table2 : Subsystem
  Lqd Lookup Table1 : Subsystem
  Lqq Lookup Table : Subsystem
  M_Mi : hdlmdlgenlib/Buffer
  Product11 : Subsystem
      mask Display: disp('NFP\nmul');
  Product111 : Subsystem
      mask Display: disp('NFP\nmul');
  Product12 : Subsystem
      mask Display: disp('NFP\nmul');
  Product121 : Subsystem
      mask Display: disp('NFP\nmul');
  Product13 : Subsystem
      mask Display: disp('NFP\nmul');
  Product2 : Subsystem
      mask Display: disp('NFP\nmul');
  Product21 : Subsystem
      mask Display: disp('NFP\nmul');
  Product3 : Subsystem
      mask Display: disp('NFP\nmul');
  Product31 : Subsystem
      mask Display: disp('NFP\nmul');
  Product4 : Subsystem
      mask Display: disp('NFP\nmul');
  Product41 : Subsystem
      mask Display: disp('NFP\nmul');
  Product9 : Subsystem
      mask Display: disp('NFP\nmul');
  Product91 : Subsystem
      mask Display: disp('NFP\nmul');
  Sign1 : Subsystem
      mask Display: disp('NFP\nsignum');
  Sum : Subsystem
      mask Display: disp('NFP\nadd');
  Sum1 : Subsystem
      mask Display: disp('NFP\nadd');
  Sum3 : Subsystem
      mask Display: disp('NFP\nadd');
  Sum31 : Subsystem
      mask Display: disp('NFP\nadd');
  Sum3_stage2 : Subsystem
      mask Display: disp('NFP\nadd');
  Sum3_stage3 : Subsystem
      mask Display: disp('NFP\nadd');
  Sum3_stage4 : Subsystem
      mask Display: disp('NFP\nadd');
  Sum4_stage2 : Subsystem
      mask Display: disp('NFP\nadd');
  Sum4_stage3 : Subsystem
      mask Display: disp('NFP\nadd');
  Sum4_stage4 : Subsystem
      mask Display: disp('NFP\nadd');
  Sum5 : Subsystem
      mask Display: disp('NFP\nadd');
  Sum51 : Subsystem
      mask Display: disp('NFP\nadd');
  Sum52 : Subsystem
      mask Display: disp('NFP\nadd');
  Switch : Switch  Criteria=u2 ~= 0  Threshold=double(0)  OutDataTypeStr=single  SampleTime=1e-08  SaturateOnIntegerOverflow=off  InputSameDT=off
  Switch1 : Switch  Criteria=u2 ~= 0  Threshold=double(0)  OutDataTypeStr=single  SampleTime=1e-08  SaturateOnIntegerOverflow=off  InputSameDT=off
  Unit Delay : RateTransition  OutPortSampleTimeOpt=Multiple of input port sample time  OutPortSampleTimeMultiple=200
  Unit Delay1 : RateTransition  OutPortSampleTimeOpt=Multiple of input port sample time  OutPortSampleTimeMultiple=200
  crp_out_delay{,1..5} (6 alike) : Delay  DelayLength=double(1)  InitialCondition=0  SampleTime=1e-08
  delayMatch{,1..18} (19 alike) : Delay  DelayLength=double(1)  InitialCondition=0  SampleTime=1e-08
  in0_repeat : RateTransition  Integrity=off  Deterministic=off  OutPortSampleTimeOpt=Multiple of input port sample time  OutPortSampleTimeMultiple=1/200
  in10_repeat : RateTransition  Integrity=off  Deterministic=off  OutPortSampleTimeOpt=Multiple of input port sample time  OutPortSampleTimeMultiple=1/200
  in11_repeat : RateTransition  Integrity=off  Deterministic=off  OutPortSampleTimeOpt=Multiple of input port sample time  OutPortSampleTimeMultiple=1/200
  in12_repeat : RateTransition  Integrity=off  Deterministic=off  OutPortSampleTimeOpt=Multiple of input port sample time  OutPortSampleTimeMultiple=1/200
  in13_repeat : RateTransition  Integrity=off  Deterministic=off  OutPortSampleTimeOpt=Multiple of input port sample time  OutPortSampleTimeMultiple=1/200
  in1_repeat : RateTransition  Integrity=off  Deterministic=off  OutPortSampleTimeOpt=Multiple of input port sample time  OutPortSampleTimeMultiple=1/200
  in2_repeat : RateTransition  Integrity=off  Deterministic=off  OutPortSampleTimeOpt=Multiple of input port sample time  OutPortSampleTimeMultiple=1/200
  in3_repeat : RateTransition  Integrity=off  Deterministic=off  OutPortSampleTimeOpt=Multiple of input port sample time  OutPortSampleTimeMultiple=1/200
  in4_repeat : RateTransition  Integrity=off  Deterministic=off  OutPortSampleTimeOpt=Multiple of input port sample time  OutPortSampleTimeMultiple=1/200
  in5_repeat : RateTransition  Integrity=off  Deterministic=off  OutPortSampleTimeOpt=Multiple of input port sample time  OutPortSampleTimeMultiple=1/200
  in6_repeat : RateTransition  Integrity=off  Deterministic=off  OutPortSampleTimeOpt=Multiple of input port sample time  OutPortSampleTimeMultiple=1/200
  in7_repeat : RateTransition  Integrity=off  Deterministic=off  OutPortSampleTimeOpt=Multiple of input port sample time  OutPortSampleTimeMultiple=1/200
  in8_repeat : RateTransition  Integrity=off  Deterministic=off  OutPortSampleTimeOpt=Multiple of input port sample time  OutPortSampleTimeMultiple=1/200
  in9_repeat : RateTransition  Integrity=off  Deterministic=off  OutPortSampleTimeOpt=Multiple of input port sample time  OutPortSampleTimeMultiple=1/200
  mux : Mux
  psi_d : hdlmdlgenlib/Buffer
  psi_q : hdlmdlgenlib/Buffer
  reset_in : Switch  Criteria=u2 ~= 0  Threshold=double(0)  OutDataTypeStr=single  SampleTime=1e-08  SaturateOnIntegerOverflow=off  InputSameDT=off
  reset_in1 : Switch  Criteria=u2 ~= 0  Threshold=double(0)  OutDataTypeStr=single  SampleTime=1e-08  SaturateOnIntegerOverflow=off  InputSameDT=off
  reset_in2 : Switch  Criteria=u2 ~= 0  Threshold=double(0)  OutDataTypeStr=single  SampleTime=1e-08  SaturateOnIntegerOverflow=off  InputSameDT=off
  reset_out : Switch  Criteria=u2 ~= 0  Threshold=double(0)  OutDataTypeStr=single  SampleTime=1e-08  SaturateOnIntegerOverflow=off  InputSameDT=off
  reset_out1 : Switch  Criteria=u2 ~= 0  Threshold=double(0)  OutDataTypeStr=single  SampleTime=1e-08  SaturateOnIntegerOverflow=off  InputSameDT=off
  reset_out2 : Switch  Criteria=u2 ~= 0  Threshold=double(0)  OutDataTypeStr=single  SampleTime=1e-08  SaturateOnIntegerOverflow=off  InputSameDT=off
  t : RateTransition  OutPortSampleTimeOpt=Multiple of input port sample time  OutPortSampleTimeMultiple=200
  t1 : Demux
  t2 : hdlmdlgenlib/Buffer
  t3 : hdlmdlgenlib/Buffer
  outputs : Outport  SampleTime=2e-06
  wires:
  reset_integrators/1 -> in1_repeat/1
  simulate_mechanical/1 -> in4_repeat/1
  reciprocal_J/1 -> in6_repeat/1
  mu/1 -> in0_repeat/1
  M_n0/1 -> in13_repeat/1
  R1/1 -> in9_repeat/1
  polepairs/1 -> in12_repeat/1
  inputs/1 -> in8_repeat/1
  t/1 -> outputs/1
  in0_repeat/1 -> Product121/1(In1)
  in1_repeat/1 -> delayMatch18/1, delayMatch12/1, delayMatch8/1, reset_out1/2, reset_out2/2, reset_out/2
  in4_repeat/1 -> Switch/2, Switch1/2
  in6_repeat/1 -> delayMatch16/1
  in8_repeat/1 -> t1/1
  in9_repeat/1 -> Product4/1(In1), Product9/2(In2)
  in12_repeat/1 -> Product13/2(In2), delayMatch2/1
  in13_repeat/1 -> delayMatch13/1
  mux/1 -> t/1
  Delay1_lowered/1 -> in11_repeat/1
  in11_repeat/1 -> reset_out2/3
  Unit Delay1/1 -> in10_repeat/1
  in10_repeat/1 -> delayMatch6/1
  Delay/1 -> in7_repeat/1
  in7_repeat/1 -> Sum1/1(In1)
  Delay1_lowered1/1 -> in5_repeat/1
  in5_repeat/1 -> reset_out1/3
  Unit Delay/1 -> in3_repeat/1
  in3_repeat/1 -> delayMatch9/1
  Delay1_lowered2/1 -> in2_repeat/1
  in2_repeat/1 -> reset_out/3
  crp_out_delay/1 -> Delay/1
  crp_out_delay1/1 -> Unit Delay/1
  crp_out_delay2/1 -> Delay1_lowered/1
  crp_out_delay3/1 -> Unit Delay1/1
  crp_out_delay4/1 -> Delay1_lowered2/1
  crp_out_delay5/1 -> Delay1_lowered1/1
  Data Type Conversion16/1 -> mux/3
  Initial_Val/1 -> reset_out/1, reset_in/1
  reset_in/1 -> crp_out_delay4/1
  Gain7/1(Out1) -> Sum5/1(In1)
  Lqq Lookup Table/1(Out1) -> Divide1/2(In2)
  Divide1/1(Out1) -> Gain7/2(In2), crp_out_delay3/1
  Lqd Lookup Table1/1(Out1) -> Product11/2(In2)
  psi_d/1 -> Product31/1(In1)
  Flux_d Lookup Table/1(Out1) -> Product2/1(In1), psi_d/1
  Product2/1(Out1) -> Sum4_stage3/2(In2)
  delayMatch5/1 -> mux/4
  Switch1/1 -> Data Type Conversion17/1
  delayMatch17/1 -> Sum3/2(In2)
  Initial_Val1/1 -> reset_out1/1, reset_in1/1
  reset_in1/1 -> crp_out_delay5/1
  delayMatch15/1 -> Sum3_stage2/1(In1)
  delayMatch10/1 -> Sum4_stage2/1(In1)
  t1/3 -> Switch/3, Switch1/3
  t1/4 -> Sum1/2(In2)
  Ldd Lookup Table/1(Out1) -> Divide_recip/1(In1)
  Ldq Lookup Table2/1(Out1) -> Product12/1(In1)
  t2/1 -> Product9/1(In1), Flux_d Lookup Table/2(In2), Flux_q Lookup Table/2(In2), Ldd Lookup Table/2(In2), Ldq Lookup Table2/2(In2), Lqd Lookup Table1/2(In2), Lqq Lookup Table/2(In2), delayMatch/1, Data Type Conversion15/1
  Flux_q Lookup Table/1(Out1) -> Product3/2(In2), psi_q/1
  psi_q/1 -> Product21/2(In2)
  delayMatch1/1 -> Product21/1(In1)
  t3/1 -> Product4/2(In2), Flux_d Lookup Table/1(In1), Flux_q Lookup Table/1(In1), Ldd Lookup Table/1(In1), Ldq Lookup Table2/1(In1), Lqd Lookup Table1/1(In1), Lqq Lookup Table/1(In1), delayMatch1/1, Data Type Conversion11/1
  Initial_Val2/1 -> reset_out2/1, reset_in2/1
  reset_in2/1 -> crp_out_delay2/1
  Gain71/1(Out1) -> Sum51/1(In1)
  Divide/1(Out1) -> Gain71/2(In2), crp_out_delay1/1
  Product3/1(Out1) -> Sum3_stage4/2(In2)
  Switch/1 -> Product13/1(In1)
  delayMatch14/1 -> Product41/2(In2)
  M_Mi/1 -> Sum/1(In1), Data Type Conversion16/1
  Product91/1(Out1) -> M_Mi/1
  Factor/1(Out1) -> Product91/1(In1)
  delayMatch/1 -> Product31/2(In2)
  delayMatch4/1 -> mux/2
  delayMatch9/1 -> Product11/1(In1)
  delayMatch6/1 -> Product12/2(In2)
  t1/1 -> delayMatch15/1
  t1/2 -> delayMatch10/1
  Gain7_const/1 -> Gain7/1(In1)
  Gain_const/1 -> Gain/1(In1)
  Gain7_const1/1 -> Gain71/1(In1)
  Factor_const/1 -> Factor/1(In1)
  delayMatch18/1 -> reset_in1/2
  delayMatch16/1 -> Product111/1(In1)
  delayMatch13/1 -> Sum52/2(In2)
  Data Type Conversion11/1 -> delayMatch3/1
  Data Type Conversion15/1 -> delayMatch4/1
  Data Type Conversion17/1 -> delayMatch5/1
  reset_out2/1 -> t3/1, delayMatch7/1
  reset_out/1 -> t2/1, delayMatch11/1
  Sum5/1(Out1) -> reset_in/3
  Product11/1(Out1) -> Sum4_stage2/2(In2)
  Sum3/1(Out1) -> reset_in1/3
  Product111/1(Out1) -> Gain/2(In2)
  Sum1/1(Out1) -> Product111/2(In2)
  Sum4_stage2/1(Out1) -> Sum4_stage3/1(In1)
  Sum4_stage3/1(Out1) -> Sum4_stage4/1(In1)
  Sum4_stage4/1(Out1) -> Divide1/1(In1)
  Product9/1(Out1) -> Sum4_stage4/2(In2)
  Product12/1(Out1) -> Sum3_stage3/2(In2)
  Product21/1(Out1) -> Sum31/2(In2)
  Product4/1(Out1) -> Sum3_stage2/2(In2)
  Sum51/1(Out1) -> reset_in2/3
  Divide_recip/1(Out1) -> Divide/2(In2)
  Sum3_stage2/1(Out1) -> Sum3_stage3/1(In1)
  Sum3_stage3/1(Out1) -> Sum3_stage4/1(In1)
  Sum3_stage4/1(Out1) -> Divide/1(In1)
  Product13/1(Out1) -> Product3/1(In1), Product2/2(In2)
  Sign1/1(Out1) -> delayMatch14/1
  Abs/1(Out1) -> Product121/2(In2)
  Product121/1(Out1) -> Sum52/1(In1)
  Sum52/1(Out1) -> Product41/1(In1)
  Product41/1(Out1) -> Sum/2(In2)
  Sum/1(Out1) -> crp_out_delay/1
  Sum31/1(Out1) -> Factor/2(In2)
  Product31/1(Out1) -> Sum31/1(In1)
  Gain/1(Out1) -> Sum3/1(In1)
  delayMatch2/1 -> Product91/2(In2)
  delayMatch3/1 -> mux/1
  delayMatch7/1 -> Sum51/2(In2)
  delayMatch8/1 -> reset_in2/2
  delayMatch11/1 -> Sum5/2(In2)
  delayMatch12/1 -> reset_in/2
  reset_out1/1 -> delayMatch17/1, Abs/1(In1), Sign1/1(In1), Switch/1, Switch1/1

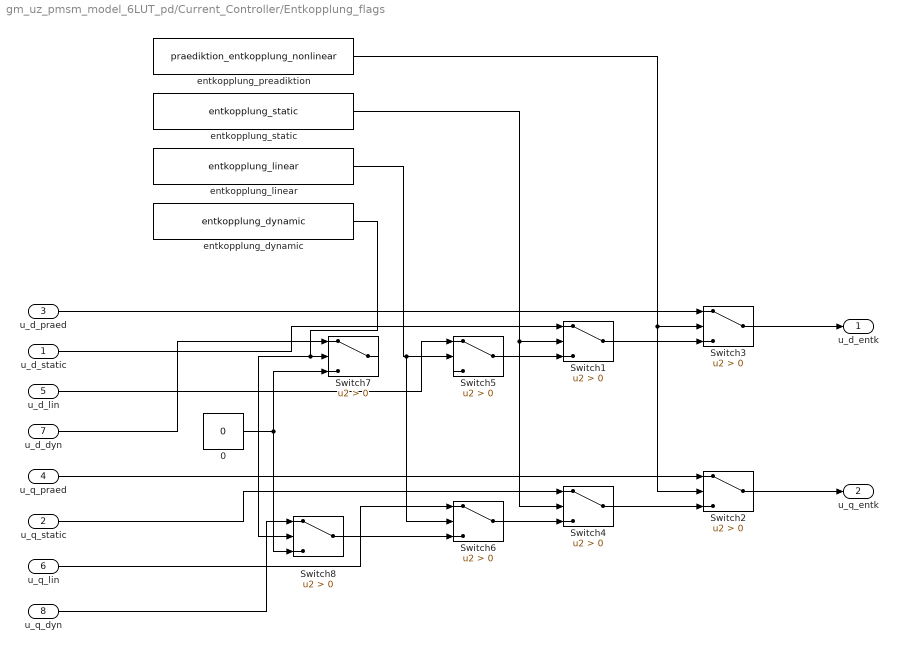
== system gm_uz_pmsm_model_6LUT_pd/Current_Controller/Entkopplung_flags ==
  u_d_static : Inport
  u_q_static : Inport  Port=2
  u_d_praed : Inport  Port=3
  u_q_praed : Inport  Port=4
  u_d_lin : Inport  Port=5
  u_q_lin : Inport  Port=6
  u_d_dyn : Inport  Port=7
  u_q_dyn : Inport  Port=8
  0 : Constant  Value=0
  Switch{1..8} (8 alike) : Switch  Criteria=u2 > Threshold  SaturateOnIntegerOverflow=off  InputSameDT=off
  entkopplung_dynamic : Constant  Value=entkopplung_dynamic
  entkopplung_linear : Constant  Value=entkopplung_linear
  entkopplung_preadiktion : Constant  Value=praediktion_entkopplung_nonlinear
  entkopplung_static : Constant  Value=entkopplung_static
  u_d_entk : Outport
  u_q_entk : Outport  Port=2
  wires:
  u_q_dyn/1 -> Switch8/1
  Switch8/1 -> Switch6/3
  u_d_dyn/1 -> Switch7/1
  u_q_lin/1 -> Switch6/1
  u_q_static/1 -> Switch4/1
  Switch6/1 -> Switch4/3
  0/1 -> Switch7/3, Switch8/3
  entkopplung_dynamic/1 -> Switch7/2, Switch8/2
  entkopplung_linear/1 -> Switch5/2, Switch6/2
  Switch5/1 -> Switch1/3
  u_d_lin/1 -> Switch5/1
  u_d_static/1 -> Switch1/1
  entkopplung_static/1 -> Switch1/2, Switch4/2
  u_q_praed/1 -> Switch2/1
  Switch2/1 -> u_q_entk/1
  u_d_praed/1 -> Switch3/1
  Switch1/1 -> Switch3/3
  entkopplung_preadiktion/1 -> Switch3/2, Switch2/2
  Switch4/1 -> Switch2/3
  Switch3/1 -> u_d_entk/1

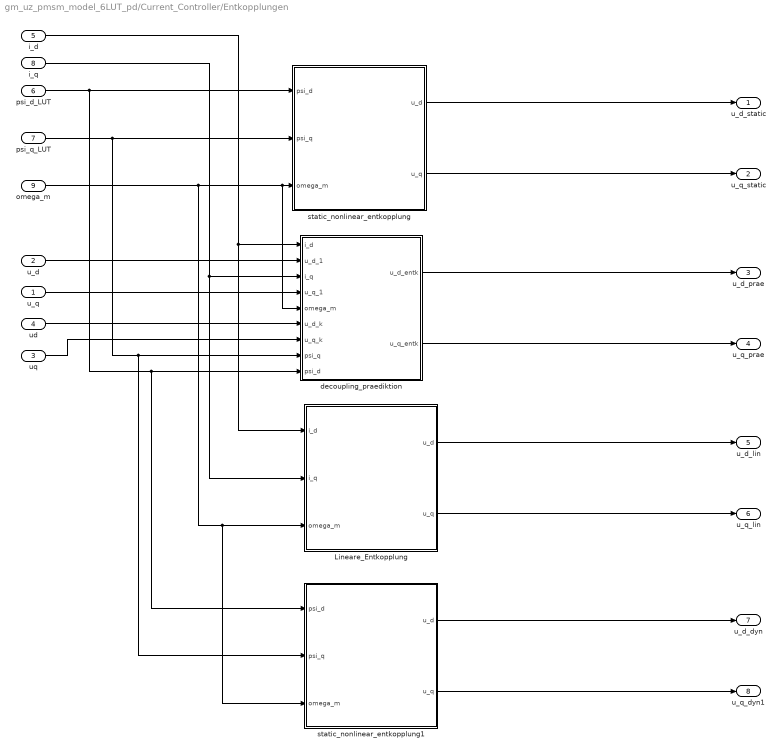
== system gm_uz_pmsm_model_6LUT_pd/Current_Controller/Entkopplungen ==
  u_q : Inport
  u_d : Inport  Port=2
  uq : Inport  Port=3
  ud : Inport  Port=4
  i_d : Inport  Port=5
  psi_d_LUT : Inport  Port=6
  psi_q_LUT : Inport  Port=7
  i_q : Inport  Port=8
  omega_m : Inport  Port=9
  Lineare_Entkopplung : Subsystem
  decoupling_praediktion : Subsystem
  static_nonlinear_entkopplung : Subsystem
  static_nonlinear_entkopplung1 : Subsystem
  u_d_static : Outport
  u_q_static : Outport  Port=2
  u_d_prae : Outport  Port=3
  u_q_prae : Outport  Port=4
  u_d_lin : Outport  Port=5
  u_q_lin : Outport  Port=6
  u_d_dyn : Outport  Port=7
  u_q_dyn1 : Outport  Port=8
  wires:
  static_nonlinear_entkopplung1/2(u_q) -> u_q_dyn1/1
  static_nonlinear_entkopplung1/1(u_d) -> u_d_dyn/1
  decoupling_praediktion/2(u_q_entk) -> u_q_prae/1
  Lineare_Entkopplung/2(u_q) -> u_q_lin/1
  decoupling_praediktion/1(u_d_entk) -> u_d_prae/1
  static_nonlinear_entkopplung/2(u_q) -> u_q_static/1
  Lineare_Entkopplung/1(u_d) -> u_d_lin/1
  static_nonlinear_entkopplung/1(u_d) -> u_d_static/1
  u_d/1 -> decoupling_praediktion/2(u_d_1)
  uq/1 -> decoupling_praediktion/7(u_q_k)
  ud/1 -> decoupling_praediktion/6(u_d_k)
  i_q/1 -> decoupling_praediktion/3(i_q), Lineare_Entkopplung/2(i_q)
  i_d/1 -> decoupling_praediktion/1(i_d), Lineare_Entkopplung/1(i_d)
  u_q/1 -> decoupling_praediktion/4(u_q_1)
  psi_q_LUT/1 -> static_nonlinear_entkopplung/2(psi_q), decoupling_praediktion/8(psi_q), static_nonlinear_entkopplung1/2(psi_q)
  omega_m/1 -> decoupling_praediktion/5(omega_m), static_nonlinear_entkopplung/3(omega_m), Lineare_Entkopplung/3(omega_m), static_nonlinear_entkopplung1/3(omega_m)
  psi_d_LUT/1 -> decoupling_praediktion/9(psi_d), static_nonlinear_entkopplung1/1(psi_d), static_nonlinear_entkopplung/1(psi_d)
